simulink model "open_loop_motor_model"  (R2022b)
settings: Solver=ode45  StartTime=0.0  StopTime=20  RelTol=1e-3
InitFcn:
  | Va=220
  | Vf=300
  | Jm=0.117
  | Bm=0.001
  | La=16.2e-3
  | Lf=71.47
  | Tl=50
  | Kb=0.699
  | Rf=180
  | Ra=2
libraries: spspowerguiLib x1
settings Model: Creator=David Ugochukwu  LastModifiedBy=ugochukwu
settings SolverCC: AlgebraicLoopSolver=TrustRegion
settings DataIOCC: LimitDataPoints=on  SaveFormat=Array  ReturnWorkspaceOutputs=off
settings OptimizationCC: BlockReduction=off  BooleanDataType=off  LifeSpan=inf
settings DebuggingCC: SaveWithParameterizedLinksMsg=none  UnderspecifiedInitializationDetection=Classic  MergeDetectMultiDrivingBlocksExec=none  SignalResolutionControl=TryResolveAllWithWarning  UnconnectedInputMsg=warning  UnconnectedOutputMsg=warning  UnconnectedLineMsg=warning  SFUnexpectedBacktrackingDiag=warning  SFNoUnconditionalDefaultTransitionDiag=warning  SFExecutionAtInitializationDiag=none  SFMachineParentedDataDiag=warning  ArithmeticOperatorsInVariantConditions=warning
settings HardwareCC: ProdBitPerPointer=32  ProdBitPerSizeT=32  ProdBitPerPtrDiffT=32  ProdLargestAtomicFloat=None  ProdIntDivRoundTo=Undefined  ProdEndianess=Unspecified  ProdWordSize=32  ProdHWDeviceType=32-bit Generic  TargetUnknown=on
settings ModelReferenceCC: EnableRefExpFcnMdlSchedulingChecks=on  PropagateSignalLabelsOutOfModel=off
settings SFSimCC: SimUseLocalCustomCode=off  CustomCodeUndefinedFunction=UseInterfaceOnly
settings RTWCC: RTWUseLocalCustomCode=off
settings CodeAppCC: StateflowObjectComments=on
settings GRTTargetCC: TargetLangStandard=C89/C90 (ANSI)
settings ConfigComp: CovMetricSettings=dw  CovSaveCumulativeToWorkspaceVar=on  CovSaveSingleToWorkspaceVar=on  CovExternalEMLEnable=off  CovSFcnEnable=off

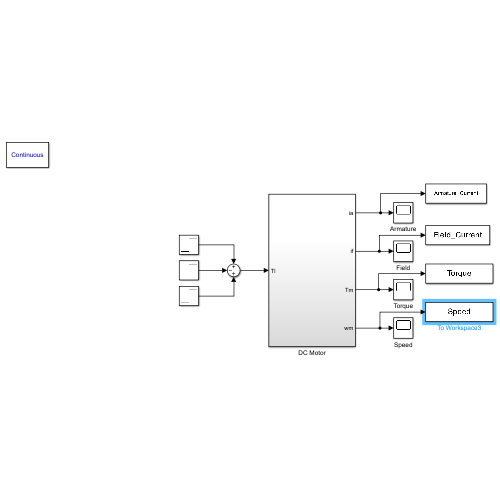
[thumbnail: Simulink's stored preview of the top-level diagram]
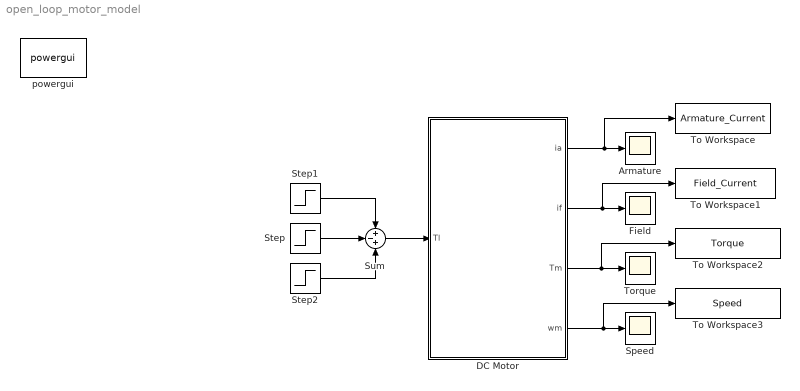
== system open_loop_motor_model ==
  Armature : Scope
  DC Motor : Subsystem
  Field : Scope
  Speed : Scope
  Step : Step  Time=9  After=20  SampleTime=0
  Step1 : Step  Time=6  After=50  SampleTime=0
  Step2 : Step  Time=13  After=70  SampleTime=0
  Sum : Sum  Inputs=+-+
  To Workspace : ToWorkspace  VariableName=Armature_Current  SaveFormat=Timeseries  SampleTime=-1
  To Workspace1 : ToWorkspace  VariableName=Field_Current  SaveFormat=Timeseries  SampleTime=-1
  To Workspace2 : ToWorkspace  VariableName=Torque  SaveFormat=Timeseries  SampleTime=-1
  To Workspace3 : ToWorkspace  VariableName=Speed  SaveFormat=Timeseries  SampleTime=-1
  Torque : Scope
  powergui : spspowerguiLib/powergui  Priority=1  SimulationMode=Continuous  SampleTime=50e-6  frequency=60  Iterations=50  frequencyindice=60  Pbase=100e6  ErrMax=1e-4  UnitsV=kV  UnitsW=MW  buscounter=0  FunctionMessages=off  echomessages=off  EnableUseOfTLC=off  CurrentSourceSwitches=off  DisableSnubberDevices=off  DisableRonSwitches=off  DisableVfSwitches=off  DisplayEquations=off  AutomaticDiscreteSolvers=off  SolverType=Tustin  Interpol=off  ExternalGateDelay=off  methode=off  Ts=0  x0status=blocks  SPID=off  SwTol=0  HookPort=off  NonlinearTolerance=1e-4  nMaxIteration=100  ContinueOnMaxIteration=off  RestoreLinks=warning  ResistiveCurrentMeasurement=off  Frange=[0:2:500]  Ylog=off  Xlog=on  ShowGrid=off  save=off  variable=ZData  structure=0  ZoomFFT=off  StartTime=0.0  cycles=1  DisplayStyle=1  fundamental=60  FreqAxis=off  MaxFrequency=1000  frequencyindicesteady=1  RmsSteady=1  display=off
  wires:
  DC Motor/1(ia) -> To Workspace/1, Armature/1
  DC Motor/2(if) -> To Workspace1/1, Field/1
  DC Motor/3(Tm) -> To Workspace2/1, Torque/1
  DC Motor/4(wm) -> To Workspace3/1, Speed/1
  Step1/1 -> Sum/1
  Step/1 -> Sum/2
  Sum/1 -> DC Motor/1(Tl)
  Step2/1 -> Sum/3

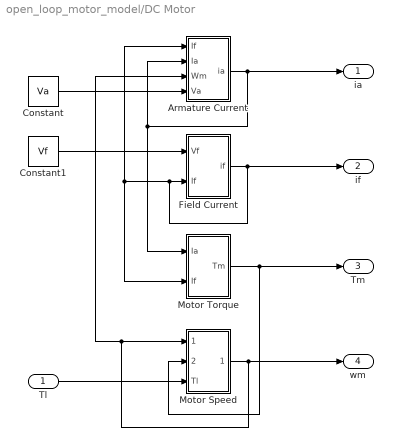
== system open_loop_motor_model/DC Motor ==
  Tl : Inport
  Armature Current : Subsystem
  Constant : Constant  Value=Va
  Constant1 : Constant  Value=Vf
  Field Current : Subsystem
  Motor Speed : Subsystem
  Motor Torque : Subsystem
  ia : Outport  VectorParamsAs1DForOutWhenUnconnected=off
  if : Outport  Port=2  VectorParamsAs1DForOutWhenUnconnected=off
  Tm : Outport  Port=3  VectorParamsAs1DForOutWhenUnconnected=off
  wm : Outport  Port=4  VectorParamsAs1DForOutWhenUnconnected=off
  wires:
  Constant1/1 -> Field Current/1(Vf)
  Motor Speed/1(Wm) -> wm/1, Armature Current/3(Wm), Motor Speed/1(wm)
  Armature Current/1(ia) -> ia/1, Motor Torque/1(Ia), Armature Current/2(Ia)
  Field Current/1(if) -> if/1, Motor Torque/2(If), Armature Current/1(If), Field Current/2(If)
  Motor Torque/1(Tm) -> Tm/1, Motor Speed/2(Tm)
  Constant/1 -> Armature Current/4(Va)
  Tl/1 -> Motor Speed/3(Tl)

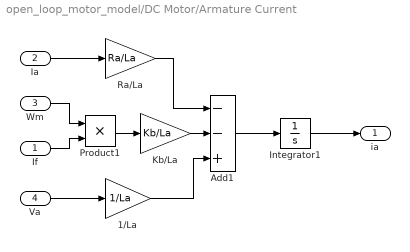
== system open_loop_motor_model/DC Motor/Armature Current ==
  If : Inport
  Ia : Inport  Port=2
  Wm : Inport  Port=3
  Va : Inport  Port=4
  1/La : Gain  Gain=1/La
  Add1 : Sum  Inputs=--+
  Integrator1 : Integrator
  Kb/La : Gain  Gain=Kb/La
  Product1 : Product
  Ra/La : Gain  Gain=Ra/La
  ia : Outport  VectorParamsAs1DForOutWhenUnconnected=off
  wires:
  Ia/1 -> Ra/La/1
  Va/1 -> 1/La/1
  Kb/La/1 -> Add1/2
  1/La/1 -> Add1/3
  Add1/1 -> Integrator1/1
  Integrator1/1 -> ia/1
  Product1/1 -> Kb/La/1
  Ra/La/1 -> Add1/1
  If/1 -> Product1/2
  Wm/1 -> Product1/1

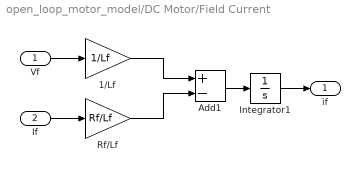
== system open_loop_motor_model/DC Motor/Field Current ==
  Vf : Inport
  If : Inport  Port=2
  1/Lf : Gain  Gain=1/Lf
  Add1 : Sum  Inputs=+-
  Integrator1 : Integrator
  Rf/Lf : Gain  Gain=Rf/Lf
  if : Outport  VectorParamsAs1DForOutWhenUnconnected=off
  wires:
  Vf/1 -> 1/Lf/1
  Rf/Lf/1 -> Add1/2
  1/Lf/1 -> Add1/1
  If/1 -> Rf/Lf/1
  Integrator1/1 -> if/1
  Add1/1 -> Integrator1/1

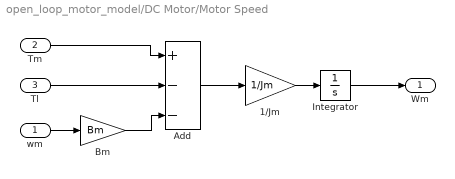
== system open_loop_motor_model/DC Motor/Motor Speed ==
  wm : Inport
  Tm : Inport  Port=2
  Tl : Inport  Port=3
  1/Jm : Gain  Gain=1/Jm
  Add : Sum  Inputs=+--
  Bm : Gain  Gain=Bm
  Integrator : Integrator
  Wm : Outport  VectorParamsAs1DForOutWhenUnconnected=off
  wires:
  1/Jm/1 -> Integrator/1
  Tl/1 -> Add/2
  Tm/1 -> Add/1
  Add/1 -> 1/Jm/1
  Integrator/1 -> Wm/1
  Bm/1 -> Add/3
  wm/1 -> Bm/1

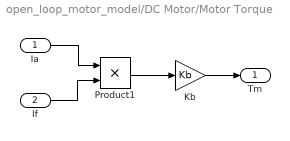
== system open_loop_motor_model/DC Motor/Motor Torque ==
  Ia : Inport
  If : Inport  Port=2
  Kb : Gain  Gain=Kb
  Product1 : Product
  Tm : Outport  VectorParamsAs1DForOutWhenUnconnected=off
  wires:
  If/1 -> Product1/2
  Product1/1 -> Kb/1
  Kb/1 -> Tm/1
  Ia/1 -> Product1/1
